simulink model "final_upfc_400kv_wavelet_windfarm_q"  (R2021a)
settings: Solver=VariableStepAuto  StartTime=0.0  StopTime=0.5  RelTol=1e-3
values from neighbouring files (symbols this model uses):
  Ts = 0.00005    (= 5e-05)    [differential_wavelet_with_wind_farm_400.m]
undefined symbols (not defined in the file or in its folder): D11, Delta, DiscIntNeverNeededParam, find_system, level
libraries: powerlib_extras x76, spsThreePhaseVIMeasurementLib x11, simulink_extras x8, spsThreeLevelBridgeLib x8, spsVoltageMeasurementLib x8, spsZigzagPhaseShiftingTransformerLib x8, spsCurrentMeasurementLib x6, spsSeriesRLCBranchLib x5, spsThreePhasePISectionLineLib x5, spsThreePhaseFaultLib x4, spsThreePhaseTransformerTwoWindingsLib x2, spsMultimeterLib x2
(part 7 of 9)

== system final_upfc_400kv_wavelet_windfarm_q/UPFC Controller/SE Control (UPFC)/Firing Pulses Generator/Bridge 1Y /Phase C ==
  note: |
      | |
      | |
      | [Q1]
      | |
      | |
  note: |
      | |
      | [Q2]
      | |
      | |
  note: |
      | |
      | [Q3]
      | |
      | |
  note: |
      | |
      | [G4]
      | |
      | |
      | |
  note: --------[D_NP]---------
  note: --------[D-NN]---------
  note: ---------- A
  note: |
      | |
      | |
      | |
      | |
      | |
      | |
      | |
      | |
      | |
      | |
  note: N -------
  note: - Vdc -------------------------------
  note: + Vdc -------------------------------
  note: Q4,Q1
  note: Q2,Q3
  note: Q1,Q2,Q3,Q4
  note: |
      | |
      | |
      | |
      | |
      | |
      | |
      | |
      | |
      | |
      | |
  note: |
      | |
      | |
      | |
      | |
      | |
      | |
      | |
      | |
      | |
      | |
  note: |
      | |
      | |
      | |
      | |
      | |
      | |
      | |
      | |
      | |
      | |
  note: Pulses timing
      | ===========
  note: Normal 180deg
      | Operation
  note: Normal 180deg
      | Operation
  note: Normal 180deg
      | Operation
  note: I--------------------------------I-----------------------------I--
  note: 0
  note: 180
  note: 360
  note: ******************
  note: ******************
  note: ********************************************
  note: ******************************************
  note: Q1
  note: Q2
  note: Q3
  note: Q4
  note: |
      | |
      | |
  note: |
      | |
      | |
  note: <--Sigma-->
  wt : Inport  PortDimensions=1
  sigma : Inport  Port=2  PortDimensions=1
  D_Alpha : Inport  Port=3  PortDimensions=1
  Constant1 : Constant  Value=[0 -pi]
  Constant2 : Constant  Value=2*pi
  Constant3 : Constant  Value=0
  Constant8 : Constant  Value=pi
  Constant9 : Constant  Value=pi
  Deg->Rad2 : Gain  Gain=0.5  SaturateOnIntegerOverflow=on  OutDataTypeStr=Inherit: Same as input  ParamDataTypeStr=Inherit: Same as input
  Deg->Rad3 : Gain  Gain=-1  SaturateOnIntegerOverflow=on  OutDataTypeStr=Inherit: Same as input  ParamDataTypeStr=Inherit: Same as input
  Gain3 : Gain  Gain=2  SaturateOnIntegerOverflow=on  OutDataTypeStr=Inherit: Same as input  ParamDataTypeStr=Inherit: Same as input
  Logical Operator : Logic
  Logical Operator2 : Logic  Operator=NOT
  Math Function : Math  Operator=mod  SignedPower=on  SaturateOnIntegerOverflow=on
  Mux3 : Mux  Inputs=[2 2]
  Mux4 : Mux  Inputs=2
  Relational Operator : RelationalOperator  RndMeth=Nearest  InputSameDT=on
  Relational Operator1 : RelationalOperator  Operator=<  RndMeth=Nearest  InputSameDT=on
  Selector3 : Selector  InputPortWidth=4  IndexOptions=Index vector (dialog)  Indices=[4 1 2 3]  OutputSizes=1
  Sum{2,4..6} (4 alike) : Sum  InputSameDT=on  SaturateOnIntegerOverflow=on  OutDataTypeStr=Inherit: Same as first input
  Sum3 : Sum  Inputs=+-  InputSameDT=on  SaturateOnIntegerOverflow=on  OutDataTypeStr=Inherit: Same as first input
  Pulses : Outport
  wires:
  Constant1/1 -> Sum2/2
  Constant3/1 -> Relational Operator/2
  Relational Operator/1 -> Logical Operator/1
  Relational Operator1/1 -> Logical Operator/2
  Constant9/1 -> Sum3/1
  sigma/1 -> Sum3/2
  Sum3/1 -> Deg->Rad2/1
  Deg->Rad2/1 -> Sum4/1, Gain3/1  "Beta"
  Constant8/1 -> Sum6/2
  Sum6/1 -> Relational Operator1/2
  Sum2/1 -> Sum4/2
  Sum4/1 -> Math Function/1
  Logical Operator/1 -> Logical Operator2/1, Mux3/1
  Logical Operator2/1 -> Mux3/2
  Mux3/1 -> Selector3/1
  Selector3/1 -> Pulses/1
  Gain3/1 -> Sum6/1
  Math Function/1 -> Relational Operator1/1, Relational Operator/1
  Mux4/1 -> Sum5/2
  Deg->Rad3/1 -> Mux4/2
  D_Alpha/1 -> Deg->Rad3/1, Mux4/1
  wt/1 -> Sum5/1  "wt"
  Sum5/1 -> Sum2/1  "theta"
  Constant2/1 -> Math Function/2

== system final_upfc_400kv_wavelet_windfarm_q/UPFC Controller/SE Control (UPFC)/Firing Pulses Generator/Bridge 2D/Phase A ==
  note: <--Sigma-->
  note: |
      | |
      | |
  note: |
      | |
      | |
  note: Q4
  note: Q3
  note: Q2
  note: Q1
  note: ******************************************
  note: ********************************************
  note: ******************
  note: ******************
  note: 360
  note: 180
  note: 0
  note: I--------------------------------I-----------------------------I--
  note: Normal 180deg
      | Operation
  note: Normal 180deg
      | Operation
  note: Normal 180deg
      | Operation
  note: Pulses timing
      | ===========
  note: |
      | |
      | |
      | |
      | |
      | |
      | |
      | |
      | |
      | |
      | |
  note: |
      | |
      | |
      | |
      | |
      | |
      | |
      | |
      | |
      | |
      | |
  note: |
      | |
      | |
      | |
      | |
      | |
      | |
      | |
      | |
      | |
      | |
  note: Q1,Q2,Q3,Q4
  note: Q2,Q3
  note: Q4,Q1
  note: + Vdc -------------------------------
  note: - Vdc -------------------------------
  note: N -------
  note: |
      | |
      | |
      | |
      | |
      | |
      | |
      | |
      | |
      | |
      | |
  note: ---------- A
  note: --------[D-NN]---------
  note: --------[D_NP]---------
  note: |
      | |
      | [G4]
      | |
      | |
      | |
  note: |
      | |
      | [Q3]
      | |
      | |
  note: |
      | |
      | [Q2]
      | |
      | |
  note: |
      | |
      | |
      | [Q1]
      | |
      | |
  wt : Inport  PortDimensions=1
  sigma : Inport  Port=2  PortDimensions=1
  D_Alpha : Inport  Port=3  PortDimensions=1
  Constant1 : Constant  Value=[0 -pi]
  Constant2 : Constant  Value=2*pi
  Constant3 : Constant  Value=0
  Constant8 : Constant  Value=pi
  Constant9 : Constant  Value=pi
  Deg->Rad2 : Gain  Gain=0.5  SaturateOnIntegerOverflow=on  OutDataTypeStr=Inherit: Same as input  ParamDataTypeStr=Inherit: Same as input
  Deg->Rad3 : Gain  Gain=-1  SaturateOnIntegerOverflow=on  OutDataTypeStr=Inherit: Same as input  ParamDataTypeStr=Inherit: Same as input
  Gain3 : Gain  Gain=2  SaturateOnIntegerOverflow=on  OutDataTypeStr=Inherit: Same as input  ParamDataTypeStr=Inherit: Same as input
  Logical Operator : Logic
  Logical Operator2 : Logic  Operator=NOT
  Math Function : Math  Operator=mod  SignedPower=on  SaturateOnIntegerOverflow=on
  Mux3 : Mux  Inputs=[2 2]
  Mux4 : Mux  Inputs=2
  Relational Operator : RelationalOperator  RndMeth=Nearest  InputSameDT=on
  Relational Operator1 : RelationalOperator  Operator=<  RndMeth=Nearest  InputSameDT=on
  Selector3 : Selector  InputPortWidth=4  IndexOptions=Index vector (dialog)  Indices=[4 1 2 3]  OutputSizes=1
  Sum{2,4..6} (4 alike) : Sum  InputSameDT=on  SaturateOnIntegerOverflow=on  OutDataTypeStr=Inherit: Same as first input
  Sum3 : Sum  Inputs=+-  InputSameDT=on  SaturateOnIntegerOverflow=on  OutDataTypeStr=Inherit: Same as first input
  Pulses : Outport
  wires:
  Constant2/1 -> Math Function/2
  Sum5/1 -> Sum2/1  "theta"
  wt/1 -> Sum5/1  "wt"
  D_Alpha/1 -> Mux4/1, Deg->Rad3/1
  Deg->Rad3/1 -> Mux4/2
  Mux4/1 -> Sum5/2
  Math Function/1 -> Relational Operator/1, Relational Operator1/1
  Gain3/1 -> Sum6/1
  Selector3/1 -> Pulses/1
  Mux3/1 -> Selector3/1
  Logical Operator2/1 -> Mux3/2
  Logical Operator/1 -> Mux3/1, Logical Operator2/1
  Sum4/1 -> Math Function/1
  Sum2/1 -> Sum4/2
  Sum6/1 -> Relational Operator1/2
  Constant8/1 -> Sum6/2
  Deg->Rad2/1 -> Gain3/1, Sum4/1  "Beta"
  Sum3/1 -> Deg->Rad2/1
  sigma/1 -> Sum3/2
  Constant9/1 -> Sum3/1
  Relational Operator1/1 -> Logical Operator/2
  Relational Operator/1 -> Logical Operator/1
  Constant3/1 -> Relational Operator/2
  Constant1/1 -> Sum2/2

== system final_upfc_400kv_wavelet_windfarm_q/UPFC Controller/SE Control (UPFC)/Firing Pulses Generator/Bridge 2D/Phase B ==
  note: |
      | |
      | |
      | [Q1]
      | |
      | |
  note: |
      | |
      | [Q2]
      | |
      | |
  note: |
      | |
      | [Q3]
      | |
      | |
  note: |
      | |
      | [G4]
      | |
      | |
      | |
  note: --------[D_NP]---------
  note: --------[D-NN]---------
  note: ---------- A
  note: |
      | |
      | |
      | |
      | |
      | |
      | |
      | |
      | |
      | |
      | |
  note: N -------
  note: - Vdc -------------------------------
  note: + Vdc -------------------------------
  note: Q4,Q1
  note: Q2,Q3
  note: Q1,Q2,Q3,Q4
  note: |
      | |
      | |
      | |
      | |
      | |
      | |
      | |
      | |
      | |
      | |
  note: |
      | |
      | |
      | |
      | |
      | |
      | |
      | |
      | |
      | |
      | |
  note: |
      | |
      | |
      | |
      | |
      | |
      | |
      | |
      | |
      | |
      | |
  note: Pulses timing
      | ===========
  note: Normal 180deg
      | Operation
  note: Normal 180deg
      | Operation
  note: Normal 180deg
      | Operation
  note: I--------------------------------I-----------------------------I--
  note: 0
  note: 180
  note: 360
  note: ******************
  note: ******************
  note: ********************************************
  note: ******************************************
  note: Q1
  note: Q2
  note: Q3
  note: Q4
  note: |
      | |
      | |
  note: |
      | |
      | |
  note: <--Sigma-->
  wt : Inport  PortDimensions=1
  sigma : Inport  Port=2  PortDimensions=1
  D_Alpha : Inport  Port=3  PortDimensions=1
  Constant1 : Constant  Value=[0 -pi]
  Constant2 : Constant  Value=2*pi
  Constant3 : Constant  Value=0
  Constant8 : Constant  Value=pi
  Constant9 : Constant  Value=pi
  Deg->Rad2 : Gain  Gain=0.5  SaturateOnIntegerOverflow=on  OutDataTypeStr=Inherit: Same as input  ParamDataTypeStr=Inherit: Same as input
  Deg->Rad3 : Gain  Gain=-1  SaturateOnIntegerOverflow=on  OutDataTypeStr=Inherit: Same as input  ParamDataTypeStr=Inherit: Same as input
  Gain3 : Gain  Gain=2  SaturateOnIntegerOverflow=on  OutDataTypeStr=Inherit: Same as input  ParamDataTypeStr=Inherit: Same as input
  Logical Operator : Logic
  Logical Operator2 : Logic  Operator=NOT
  Math Function : Math  Operator=mod  SignedPower=on  SaturateOnIntegerOverflow=on
  Mux3 : Mux  Inputs=[2 2]
  Mux4 : Mux  Inputs=2
  Relational Operator : RelationalOperator  RndMeth=Nearest  InputSameDT=on
  Relational Operator1 : RelationalOperator  Operator=<  RndMeth=Nearest  InputSameDT=on
  Selector3 : Selector  InputPortWidth=4  IndexOptions=Index vector (dialog)  Indices=[4 1 2 3]  OutputSizes=1
  Sum{2,4..6} (4 alike) : Sum  InputSameDT=on  SaturateOnIntegerOverflow=on  OutDataTypeStr=Inherit: Same as first input
  Sum3 : Sum  Inputs=+-  InputSameDT=on  SaturateOnIntegerOverflow=on  OutDataTypeStr=Inherit: Same as first input
  Pulses : Outport
  wires:
  Constant1/1 -> Sum2/2
  Constant3/1 -> Relational Operator/2
  Relational Operator/1 -> Logical Operator/1
  Relational Operator1/1 -> Logical Operator/2
  Constant9/1 -> Sum3/1
  sigma/1 -> Sum3/2
  Sum3/1 -> Deg->Rad2/1
  Deg->Rad2/1 -> Sum4/1, Gain3/1  "Beta"
  Constant8/1 -> Sum6/2
  Sum6/1 -> Relational Operator1/2
  Sum2/1 -> Sum4/2
  Sum4/1 -> Math Function/1
  Logical Operator/1 -> Logical Operator2/1, Mux3/1
  Logical Operator2/1 -> Mux3/2
  Mux3/1 -> Selector3/1
  Selector3/1 -> Pulses/1
  Gain3/1 -> Sum6/1
  Math Function/1 -> Relational Operator1/1, Relational Operator/1
  Mux4/1 -> Sum5/2
  Deg->Rad3/1 -> Mux4/2
  D_Alpha/1 -> Deg->Rad3/1, Mux4/1
  wt/1 -> Sum5/1  "wt"
  Sum5/1 -> Sum2/1  "theta"
  Constant2/1 -> Math Function/2

== system final_upfc_400kv_wavelet_windfarm_q/UPFC Controller/SE Control (UPFC)/Firing Pulses Generator/Bridge 2D/Phase C ==
  note: <--Sigma-->
  note: |
      | |
      | |
  note: |
      | |
      | |
  note: Q4
  note: Q3
  note: Q2
  note: Q1
  note: ******************************************
  note: ********************************************
  note: ******************
  note: ******************
  note: 360
  note: 180
  note: 0
  note: I--------------------------------I-----------------------------I--
  note: Normal 180deg
      | Operation
  note: Normal 180deg
      | Operation
  note: Normal 180deg
      | Operation
  note: Pulses timing
      | ===========
  note: |
      | |
      | |
      | |
      | |
      | |
      | |
      | |
      | |
      | |
      | |
  note: |
      | |
      | |
      | |
      | |
      | |
      | |
      | |
      | |
      | |
      | |
  note: |
      | |
      | |
      | |
      | |
      | |
      | |
      | |
      | |
      | |
      | |
  note: Q1,Q2,Q3,Q4
  note: Q2,Q3
  note: Q4,Q1
  note: + Vdc -------------------------------
  note: - Vdc -------------------------------
  note: N -------
  note: |
      | |
      | |
      | |
      | |
      | |
      | |
      | |
      | |
      | |
      | |
  note: ---------- A
  note: --------[D-NN]---------
  note: --------[D_NP]---------
  note: |
      | |
      | [G4]
      | |
      | |
      | |
  note: |
      | |
      | [Q3]
      | |
      | |
  note: |
      | |
      | [Q2]
      | |
      | |
  note: |
      | |
      | |
      | [Q1]
      | |
      | |
  wt : Inport  PortDimensions=1
  sigma : Inport  Port=2  PortDimensions=1
  D_Alpha : Inport  Port=3  PortDimensions=1
  Constant1 : Constant  Value=[0 -pi]
  Constant2 : Constant  Value=2*pi
  Constant3 : Constant  Value=0
  Constant8 : Constant  Value=pi
  Constant9 : Constant  Value=pi
  Deg->Rad2 : Gain  Gain=0.5  SaturateOnIntegerOverflow=on  OutDataTypeStr=Inherit: Same as input  ParamDataTypeStr=Inherit: Same as input
  Deg->Rad3 : Gain  Gain=-1  SaturateOnIntegerOverflow=on  OutDataTypeStr=Inherit: Same as input  ParamDataTypeStr=Inherit: Same as input
  Gain3 : Gain  Gain=2  SaturateOnIntegerOverflow=on  OutDataTypeStr=Inherit: Same as input  ParamDataTypeStr=Inherit: Same as input
  Logical Operator : Logic
  Logical Operator2 : Logic  Operator=NOT
  Math Function : Math  Operator=mod  SignedPower=on  SaturateOnIntegerOverflow=on
  Mux3 : Mux  Inputs=[2 2]
  Mux4 : Mux  Inputs=2
  Relational Operator : RelationalOperator  RndMeth=Nearest  InputSameDT=on
  Relational Operator1 : RelationalOperator  Operator=<  RndMeth=Nearest  InputSameDT=on
  Selector3 : Selector  InputPortWidth=4  IndexOptions=Index vector (dialog)  Indices=[4 1 2 3]  OutputSizes=1
  Sum{2,4..6} (4 alike) : Sum  InputSameDT=on  SaturateOnIntegerOverflow=on  OutDataTypeStr=Inherit: Same as first input
  Sum3 : Sum  Inputs=+-  InputSameDT=on  SaturateOnIntegerOverflow=on  OutDataTypeStr=Inherit: Same as first input
  Pulses : Outport
  wires:
  Constant2/1 -> Math Function/2
  Sum5/1 -> Sum2/1  "theta"
  wt/1 -> Sum5/1  "wt"
  D_Alpha/1 -> Mux4/1, Deg->Rad3/1
  Deg->Rad3/1 -> Mux4/2
  Mux4/1 -> Sum5/2
  Math Function/1 -> Relational Operator/1, Relational Operator1/1
  Gain3/1 -> Sum6/1
  Selector3/1 -> Pulses/1
  Mux3/1 -> Selector3/1
  Logical Operator2/1 -> Mux3/2
  Logical Operator/1 -> Mux3/1, Logical Operator2/1
  Sum4/1 -> Math Function/1
  Sum2/1 -> Sum4/2
  Sum6/1 -> Relational Operator1/2
  Constant8/1 -> Sum6/2
  Deg->Rad2/1 -> Gain3/1, Sum4/1  "Beta"
  Sum3/1 -> Deg->Rad2/1
  sigma/1 -> Sum3/2
  Constant9/1 -> Sum3/1
  Relational Operator1/1 -> Logical Operator/2
  Relational Operator/1 -> Logical Operator/1
  Constant3/1 -> Relational Operator/2
  Constant1/1 -> Sum2/2

== system final_upfc_400kv_wavelet_windfarm_q/UPFC Controller/SE Control (UPFC)/Firing Pulses Generator/Bridge 2Y/Phase A ==
  note: |
      | |
      | |
      | [Q1]
      | |
      | |
  note: |
      | |
      | [Q2]
      | |
      | |
  note: |
      | |
      | [Q3]
      | |
      | |
  note: |
      | |
      | [G4]
      | |
      | |
      | |
  note: --------[D_NP]---------
  note: --------[D-NN]---------
  note: ---------- A
  note: |
      | |
      | |
      | |
      | |
      | |
      | |
      | |
      | |
      | |
      | |
  note: N -------
  note: - Vdc -------------------------------
  note: + Vdc -------------------------------
  note: Q4,Q1
  note: Q2,Q3
  note: Q1,Q2,Q3,Q4
  note: |
      | |
      | |
      | |
      | |
      | |
      | |
      | |
      | |
      | |
      | |
  note: |
      | |
      | |
      | |
      | |
      | |
      | |
      | |
      | |
      | |
      | |
  note: |
      | |
      | |
      | |
      | |
      | |
      | |
      | |
      | |
      | |
      | |
  note: Pulses timing
      | ===========
  note: Normal 180deg
      | Operation
  note: Normal 180deg
      | Operation
  note: Normal 180deg
      | Operation
  note: I--------------------------------I-----------------------------I--
  note: 0
  note: 180
  note: 360
  note: ******************
  note: ******************
  note: ********************************************
  note: ******************************************
  note: Q1
  note: Q2
  note: Q3
  note: Q4
  note: |
      | |
      | |
  note: |
      | |
      | |
  note: <--Sigma-->
  wt : Inport  PortDimensions=1
  sigma : Inport  Port=2  PortDimensions=1
  D_Alpha : Inport  Port=3  PortDimensions=1
  Constant1 : Constant  Value=[0 -pi]
  Constant2 : Constant  Value=2*pi
  Constant3 : Constant  Value=0
  Constant8 : Constant  Value=pi
  Constant9 : Constant  Value=pi
  Deg->Rad2 : Gain  Gain=0.5  SaturateOnIntegerOverflow=on  OutDataTypeStr=Inherit: Same as input  ParamDataTypeStr=Inherit: Same as input
  Deg->Rad3 : Gain  Gain=-1  SaturateOnIntegerOverflow=on  OutDataTypeStr=Inherit: Same as input  ParamDataTypeStr=Inherit: Same as input
  Gain3 : Gain  Gain=2  SaturateOnIntegerOverflow=on  OutDataTypeStr=Inherit: Same as input  ParamDataTypeStr=Inherit: Same as input
  Logical Operator : Logic
  Logical Operator2 : Logic  Operator=NOT
  Math Function : Math  Operator=mod  SignedPower=on  SaturateOnIntegerOverflow=on
  Mux3 : Mux  Inputs=[2 2]
  Mux4 : Mux  Inputs=2
  Relational Operator : RelationalOperator  RndMeth=Nearest  InputSameDT=on
  Relational Operator1 : RelationalOperator  Operator=<  RndMeth=Nearest  InputSameDT=on
  Selector3 : Selector  InputPortWidth=4  IndexOptions=Index vector (dialog)  Indices=[4 1 2 3]  OutputSizes=1
  Sum{2,4..6} (4 alike) : Sum  InputSameDT=on  SaturateOnIntegerOverflow=on  OutDataTypeStr=Inherit: Same as first input
  Sum3 : Sum  Inputs=+-  InputSameDT=on  SaturateOnIntegerOverflow=on  OutDataTypeStr=Inherit: Same as first input
  Pulses : Outport
  wires:
  Constant1/1 -> Sum2/2
  Constant3/1 -> Relational Operator/2
  Relational Operator/1 -> Logical Operator/1
  Relational Operator1/1 -> Logical Operator/2
  Constant9/1 -> Sum3/1
  sigma/1 -> Sum3/2
  Sum3/1 -> Deg->Rad2/1
  Deg->Rad2/1 -> Sum4/1, Gain3/1  "Beta"
  Constant8/1 -> Sum6/2
  Sum6/1 -> Relational Operator1/2
  Sum2/1 -> Sum4/2
  Sum4/1 -> Math Function/1
  Logical Operator/1 -> Logical Operator2/1, Mux3/1
  Logical Operator2/1 -> Mux3/2
  Mux3/1 -> Selector3/1
  Selector3/1 -> Pulses/1
  Gain3/1 -> Sum6/1
  Math Function/1 -> Relational Operator1/1, Relational Operator/1
  Mux4/1 -> Sum5/2
  Deg->Rad3/1 -> Mux4/2
  D_Alpha/1 -> Deg->Rad3/1, Mux4/1
  wt/1 -> Sum5/1  "wt"
  Sum5/1 -> Sum2/1  "theta"
  Constant2/1 -> Math Function/2

== system final_upfc_400kv_wavelet_windfarm_q/UPFC Controller/SE Control (UPFC)/Firing Pulses Generator/Bridge 2Y/Phase B ==
  note: <--Sigma-->
  note: |
      | |
      | |
  note: |
      | |
      | |
  note: Q4
  note: Q3
  note: Q2
  note: Q1
  note: ******************************************
  note: ********************************************
  note: ******************
  note: ******************
  note: 360
  note: 180
  note: 0
  note: I--------------------------------I-----------------------------I--
  note: Normal 180deg
      | Operation
  note: Normal 180deg
      | Operation
  note: Normal 180deg
      | Operation
  note: Pulses timing
      | ===========
  note: |
      | |
      | |
      | |
      | |
      | |
      | |
      | |
      | |
      | |
      | |
  note: |
      | |
      | |
      | |
      | |
      | |
      | |
      | |
      | |
      | |
      | |
  note: |
      | |
      | |
      | |
      | |
      | |
      | |
      | |
      | |
      | |
      | |
  note: Q1,Q2,Q3,Q4
  note: Q2,Q3
  note: Q4,Q1
  note: + Vdc -------------------------------
  note: - Vdc -------------------------------
  note: N -------
  note: |
      | |
      | |
      | |
      | |
      | |
      | |
      | |
      | |
      | |
      | |
  note: ---------- A
  note: --------[D-NN]---------
  note: --------[D_NP]---------
  note: |
      | |
      | [G4]
      | |
      | |
      | |
  note: |
      | |
      | [Q3]
      | |
      | |
  note: |
      | |
      | [Q2]
      | |
      | |
  note: |
      | |
      | |
      | [Q1]
      | |
      | |
  wt : Inport  PortDimensions=1
  sigma : Inport  Port=2  PortDimensions=1
  D_Alpha : Inport  Port=3  PortDimensions=1
  Constant1 : Constant  Value=[0 -pi]
  Constant2 : Constant  Value=2*pi
  Constant3 : Constant  Value=0
  Constant8 : Constant  Value=pi
  Constant9 : Constant  Value=pi
  Deg->Rad2 : Gain  Gain=0.5  SaturateOnIntegerOverflow=on  OutDataTypeStr=Inherit: Same as input  ParamDataTypeStr=Inherit: Same as input
  Deg->Rad3 : Gain  Gain=-1  SaturateOnIntegerOverflow=on  OutDataTypeStr=Inherit: Same as input  ParamDataTypeStr=Inherit: Same as input
  Gain3 : Gain  Gain=2  SaturateOnIntegerOverflow=on  OutDataTypeStr=Inherit: Same as input  ParamDataTypeStr=Inherit: Same as input
  Logical Operator : Logic
  Logical Operator2 : Logic  Operator=NOT
  Math Function : Math  Operator=mod  SignedPower=on  SaturateOnIntegerOverflow=on
  Mux3 : Mux  Inputs=[2 2]
  Mux4 : Mux  Inputs=2
  Relational Operator : RelationalOperator  RndMeth=Nearest  InputSameDT=on
  Relational Operator1 : RelationalOperator  Operator=<  RndMeth=Nearest  InputSameDT=on
  Selector3 : Selector  InputPortWidth=4  IndexOptions=Index vector (dialog)  Indices=[4 1 2 3]  OutputSizes=1
  Sum{2,4..6} (4 alike) : Sum  InputSameDT=on  SaturateOnIntegerOverflow=on  OutDataTypeStr=Inherit: Same as first input
  Sum3 : Sum  Inputs=+-  InputSameDT=on  SaturateOnIntegerOverflow=on  OutDataTypeStr=Inherit: Same as first input
  Pulses : Outport
  wires:
  Constant2/1 -> Math Function/2
  Sum5/1 -> Sum2/1  "theta"
  wt/1 -> Sum5/1  "wt"
  D_Alpha/1 -> Mux4/1, Deg->Rad3/1
  Deg->Rad3/1 -> Mux4/2
  Mux4/1 -> Sum5/2
  Math Function/1 -> Relational Operator/1, Relational Operator1/1
  Gain3/1 -> Sum6/1
  Selector3/1 -> Pulses/1
  Mux3/1 -> Selector3/1
  Logical Operator2/1 -> Mux3/2
  Logical Operator/1 -> Mux3/1, Logical Operator2/1
  Sum4/1 -> Math Function/1
  Sum2/1 -> Sum4/2
  Sum6/1 -> Relational Operator1/2
  Constant8/1 -> Sum6/2
  Deg->Rad2/1 -> Gain3/1, Sum4/1  "Beta"
  Sum3/1 -> Deg->Rad2/1
  sigma/1 -> Sum3/2
  Constant9/1 -> Sum3/1
  Relational Operator1/1 -> Logical Operator/2
  Relational Operator/1 -> Logical Operator/1
  Constant3/1 -> Relational Operator/2
  Constant1/1 -> Sum2/2

== system final_upfc_400kv_wavelet_windfarm_q/UPFC Controller/SE Control (UPFC)/Firing Pulses Generator/Bridge 2Y/Phase C ==
  note: |
      | |
      | |
      | [Q1]
      | |
      | |
  note: |
      | |
      | [Q2]
      | |
      | |
  note: |
      | |
      | [Q3]
      | |
      | |
  note: |
      | |
      | [G4]
      | |
      | |
      | |
  note: --------[D_NP]---------
  note: --------[D-NN]---------
  note: ---------- A
  note: |
      | |
      | |
      | |
      | |
      | |
      | |
      | |
      | |
      | |
      | |
  note: N -------
  note: - Vdc -------------------------------
  note: + Vdc -------------------------------
  note: Q4,Q1
  note: Q2,Q3
  note: Q1,Q2,Q3,Q4
  note: |
      | |
      | |
      | |
      | |
      | |
      | |
      | |
      | |
      | |
      | |
  note: |
      | |
      | |
      | |
      | |
      | |
      | |
      | |
      | |
      | |
      | |
  note: |
      | |
      | |
      | |
      | |
      | |
      | |
      | |
      | |
      | |
      | |
  note: Pulses timing
      | ===========
  note: Normal 180deg
      | Operation
  note: Normal 180deg
      | Operation
  note: Normal 180deg
      | Operation
  note: I--------------------------------I-----------------------------I--
  note: 0
  note: 180
  note: 360
  note: ******************
  note: ******************
  note: ********************************************
  note: ******************************************
  note: Q1
  note: Q2
  note: Q3
  note: Q4
  note: |
      | |
      | |
  note: |
      | |
      | |
  note: <--Sigma-->
  wt : Inport  PortDimensions=1
  sigma : Inport  Port=2  PortDimensions=1
  D_Alpha : Inport  Port=3  PortDimensions=1
  Constant1 : Constant  Value=[0 -pi]
  Constant2 : Constant  Value=2*pi
  Constant3 : Constant  Value=0
  Constant8 : Constant  Value=pi
  Constant9 : Constant  Value=pi
  Deg->Rad2 : Gain  Gain=0.5  SaturateOnIntegerOverflow=on  OutDataTypeStr=Inherit: Same as input  ParamDataTypeStr=Inherit: Same as input
  Deg->Rad3 : Gain  Gain=-1  SaturateOnIntegerOverflow=on  OutDataTypeStr=Inherit: Same as input  ParamDataTypeStr=Inherit: Same as input
  Gain3 : Gain  Gain=2  SaturateOnIntegerOverflow=on  OutDataTypeStr=Inherit: Same as input  ParamDataTypeStr=Inherit: Same as input
  Logical Operator : Logic
  Logical Operator2 : Logic  Operator=NOT
  Math Function : Math  Operator=mod  SignedPower=on  SaturateOnIntegerOverflow=on
  Mux3 : Mux  Inputs=[2 2]
  Mux4 : Mux  Inputs=2
  Relational Operator : RelationalOperator  RndMeth=Nearest  InputSameDT=on
  Relational Operator1 : RelationalOperator  Operator=<  RndMeth=Nearest  InputSameDT=on
  Selector3 : Selector  InputPortWidth=4  IndexOptions=Index vector (dialog)  Indices=[4 1 2 3]  OutputSizes=1
  Sum{2,4..6} (4 alike) : Sum  InputSameDT=on  SaturateOnIntegerOverflow=on  OutDataTypeStr=Inherit: Same as first input
  Sum3 : Sum  Inputs=+-  InputSameDT=on  SaturateOnIntegerOverflow=on  OutDataTypeStr=Inherit: Same as first input
  Pulses : Outport
  wires:
  Constant1/1 -> Sum2/2
  Constant3/1 -> Relational Operator/2
  Relational Operator/1 -> Logical Operator/1
  Relational Operator1/1 -> Logical Operator/2
  Constant9/1 -> Sum3/1
  sigma/1 -> Sum3/2
  Sum3/1 -> Deg->Rad2/1
  Deg->Rad2/1 -> Sum4/1, Gain3/1  "Beta"
  Constant8/1 -> Sum6/2
  Sum6/1 -> Relational Operator1/2
  Sum2/1 -> Sum4/2
  Sum4/1 -> Math Function/1
  Logical Operator/1 -> Logical Operator2/1, Mux3/1
  Logical Operator2/1 -> Mux3/2
  Mux3/1 -> Selector3/1
  Selector3/1 -> Pulses/1
  Gain3/1 -> Sum6/1
  Math Function/1 -> Relational Operator1/1, Relational Operator/1
  Mux4/1 -> Sum5/2
  Deg->Rad3/1 -> Mux4/2
  D_Alpha/1 -> Deg->Rad3/1, Mux4/1
  wt/1 -> Sum5/1  "wt"
  Sum5/1 -> Sum2/1  "theta"
  Constant2/1 -> Math Function/2

== system final_upfc_400kv_wavelet_windfarm_q/UPFC Controller/SE Control (UPFC)/Measurement System/Voltage Measurement/Discrete Variable Frequency Mean value1 ==
  note: Pierre Giroux, Gilbert Sybille
      | Power System Simulation Laboratory
      | IREQ, Hydro-Quebc
  note: Variable frequency - Discrete Mean Value
  Freq : Inport
  In : Inport  Port=2
  Constant : Constant  Value=Vinit
  Gain : Gain  Gain=Ts  SaturateOnIntegerOverflow=on  OutDataTypeStr=Inherit: Same as input  ParamDataTypeStr=Inherit: Same as input
  Integ4 : DiscreteIntegrator  IntegratorMethod=Integration: Trapezoidal  SampleTime=Ts  ICPrevOutput=DiscIntNeverNeededParam  ICPrevScaledInput=DiscIntNeverNeededParam
  K2 : Constant  Value=Ts/2
  Number of sample/cycle : Fcn  Expr=1/(u[1]+1e-6)/Ts
  Product : Product  InputSameDT=on  SaturateOnIntegerOverflow=on  OutDataTypeStr=Inherit: Same as first input
  Product1 : Product  Inputs=*/*  InputSameDT=on  SaturateOnIntegerOverflow=on  OutDataTypeStr=Inherit: Same as first input
  Rounding Function : Rounding  Operator=round
  Step : Step  Time=1/Finit  SampleTime=Ts
  Sum3 : Sum  Inputs=-+  InputSameDT=on  SaturateOnIntegerOverflow=on  OutDataTypeStr=Inherit: Same as first input
  Sum4 : Sum  Inputs=-+  InputSameDT=on  SaturateOnIntegerOverflow=on  OutDataTypeStr=Inherit: Same as first input
  Sum5 : Sum  InputSameDT=on  SaturateOnIntegerOverflow=on  OutDataTypeStr=Inherit: Same as first input
  Sum7 : Sum  Inputs=-+  InputSameDT=on  SaturateOnIntegerOverflow=on  OutDataTypeStr=Inherit: Same as first input
  Switch : Switch  Threshold=0.5  SaturateOnIntegerOverflow=on  InputSameDT=on
  Variable Transport Delay2 : VariableTransportDelay  MaximumDelay=20e-3
  Mean : Outport
  wires:
  Product1/1 -> Sum5/2  "Correction"
  In/1 -> Product1/3, Integ4/1  "In"
  Product/1 -> Sum5/1  "Mean value"
  Variable Transport Delay2/1 -> Sum7/1
  Sum7/1 -> Product/1
  Integ4/1 -> Variable Transport Delay2/1, Sum7/2
  Freq/1 -> Product/2, Number of sample/cycle/1  "Freq"
  K2/1 -> Sum3/1
  Gain/1 -> Sum3/2
  Rounding Function/1 -> Gain/1, Product1/2, Sum4/1
  Sum4/1 -> Product1/1
  Number of sample/cycle/1 -> Rounding Function/1, Sum4/2
  Sum3/1 -> Variable Transport Delay2/2  "Delay"
  Sum5/1 -> Switch/1
  Step/1 -> Switch/2
  Constant/1 -> Switch/3
  Switch/1 -> Mean/1

== system final_upfc_400kv_wavelet_windfarm_q/UPFC Controller/SE Control (UPFC)/Measurement System/Voltage Measurement/Discrete Variable Frequency Mean value2 ==
  note: Pierre Giroux, Gilbert Sybille
      | Power System Simulation Laboratory
      | IREQ, Hydro-Quebc
  note: Variable frequency - Discrete Mean Value
  Freq : Inport
  In : Inport  Port=2
  Constant : Constant  Value=Vinit
  Gain : Gain  Gain=Ts  SaturateOnIntegerOverflow=on  OutDataTypeStr=Inherit: Same as input  ParamDataTypeStr=Inherit: Same as input
  Integ4 : DiscreteIntegrator  IntegratorMethod=Integration: Trapezoidal  SampleTime=Ts  ICPrevOutput=DiscIntNeverNeededParam  ICPrevScaledInput=DiscIntNeverNeededParam
  K2 : Constant  Value=Ts/2
  Number of sample/cycle : Fcn  Expr=1/(u[1]+1e-6)/Ts
  Product : Product  InputSameDT=on  SaturateOnIntegerOverflow=on  OutDataTypeStr=Inherit: Same as first input
  Product1 : Product  Inputs=*/*  InputSameDT=on  SaturateOnIntegerOverflow=on  OutDataTypeStr=Inherit: Same as first input
  Rounding Function : Rounding  Operator=round
  Step : Step  Time=1/Finit  SampleTime=Ts
  Sum3 : Sum  Inputs=-+  InputSameDT=on  SaturateOnIntegerOverflow=on  OutDataTypeStr=Inherit: Same as first input
  Sum4 : Sum  Inputs=-+  InputSameDT=on  SaturateOnIntegerOverflow=on  OutDataTypeStr=Inherit: Same as first input
  Sum5 : Sum  InputSameDT=on  SaturateOnIntegerOverflow=on  OutDataTypeStr=Inherit: Same as first input
  Sum7 : Sum  Inputs=-+  InputSameDT=on  SaturateOnIntegerOverflow=on  OutDataTypeStr=Inherit: Same as first input
  Switch : Switch  Threshold=0.5  SaturateOnIntegerOverflow=on  InputSameDT=on
  Variable Transport Delay2 : VariableTransportDelay  MaximumDelay=20e-3
  Mean : Outport
  wires:
  Product1/1 -> Sum5/2  "Correction"
  In/1 -> Product1/3, Integ4/1  "In"
  Product/1 -> Sum5/1  "Mean value"
  Variable Transport Delay2/1 -> Sum7/1
  Sum7/1 -> Product/1
  Integ4/1 -> Variable Transport Delay2/1, Sum7/2
  Freq/1 -> Product/2, Number of sample/cycle/1  "Freq"
  K2/1 -> Sum3/1
  Gain/1 -> Sum3/2
  Rounding Function/1 -> Gain/1, Product1/2, Sum4/1
  Sum4/1 -> Product1/1
  Number of sample/cycle/1 -> Rounding Function/1, Sum4/2
  Sum3/1 -> Variable Transport Delay2/2  "Delay"
  Sum5/1 -> Switch/1
  Step/1 -> Switch/2
  Constant/1 -> Switch/3
  Switch/1 -> Mean/1

== system final_upfc_400kv_wavelet_windfarm_q/UPFC Controller/SE Control (UPFC)/Measurement System/Voltage Measurement1/Discrete Variable Frequency Mean value1 ==
  note: Variable frequency - Discrete Mean Value
  note: Pierre Giroux, Gilbert Sybille
      | Power System Simulation Laboratory
      | IREQ, Hydro-Quebc
  Freq : Inport
  In : Inport  Port=2
  Constant : Constant  Value=Vinit
  Gain : Gain  Gain=Ts  SaturateOnIntegerOverflow=on  OutDataTypeStr=Inherit: Same as input  ParamDataTypeStr=Inherit: Same as input
  Integ4 : DiscreteIntegrator  IntegratorMethod=Integration: Trapezoidal  SampleTime=Ts  ICPrevOutput=DiscIntNeverNeededParam  ICPrevScaledInput=DiscIntNeverNeededParam
  K2 : Constant  Value=Ts/2
  Number of sample/cycle : Fcn  Expr=1/(u[1]+1e-6)/Ts
  Product : Product  InputSameDT=on  SaturateOnIntegerOverflow=on  OutDataTypeStr=Inherit: Same as first input
  Product1 : Product  Inputs=*/*  InputSameDT=on  SaturateOnIntegerOverflow=on  OutDataTypeStr=Inherit: Same as first input
  Rounding Function : Rounding  Operator=round
  Step : Step  Time=1/Finit  SampleTime=Ts
  Sum3 : Sum  Inputs=-+  InputSameDT=on  SaturateOnIntegerOverflow=on  OutDataTypeStr=Inherit: Same as first input
  Sum4 : Sum  Inputs=-+  InputSameDT=on  SaturateOnIntegerOverflow=on  OutDataTypeStr=Inherit: Same as first input
  Sum5 : Sum  InputSameDT=on  SaturateOnIntegerOverflow=on  OutDataTypeStr=Inherit: Same as first input
  Sum7 : Sum  Inputs=-+  InputSameDT=on  SaturateOnIntegerOverflow=on  OutDataTypeStr=Inherit: Same as first input
  Switch : Switch  Threshold=0.5  SaturateOnIntegerOverflow=on  InputSameDT=on
  Variable Transport Delay2 : VariableTransportDelay  MaximumDelay=20e-3
  Mean : Outport
  wires:
  Switch/1 -> Mean/1
  Constant/1 -> Switch/3
  Step/1 -> Switch/2
  Sum5/1 -> Switch/1
  Sum3/1 -> Variable Transport Delay2/2  "Delay"
  Number of sample/cycle/1 -> Sum4/2, Rounding Function/1
  Sum4/1 -> Product1/1
  Rounding Function/1 -> Sum4/1, Product1/2, Gain/1
  Gain/1 -> Sum3/2
  K2/1 -> Sum3/1
  Freq/1 -> Number of sample/cycle/1, Product/2  "Freq"
  Integ4/1 -> Sum7/2, Variable Transport Delay2/1
  Sum7/1 -> Product/1
  Variable Transport Delay2/1 -> Sum7/1
  Product/1 -> Sum5/1  "Mean value"
  In/1 -> Integ4/1, Product1/3  "In"
  Product1/1 -> Sum5/2  "Correction"

== system final_upfc_400kv_wavelet_windfarm_q/UPFC Controller/SE Control (UPFC)/Measurement System/Voltage Measurement1/Discrete Variable Frequency Mean value2 ==
  note: Variable frequency - Discrete Mean Value
  note: Pierre Giroux, Gilbert Sybille
      | Power System Simulation Laboratory
      | IREQ, Hydro-Quebc
  Freq : Inport
  In : Inport  Port=2
  Constant : Constant  Value=Vinit
  Gain : Gain  Gain=Ts  SaturateOnIntegerOverflow=on  OutDataTypeStr=Inherit: Same as input  ParamDataTypeStr=Inherit: Same as input
  Integ4 : DiscreteIntegrator  IntegratorMethod=Integration: Trapezoidal  SampleTime=Ts  ICPrevOutput=DiscIntNeverNeededParam  ICPrevScaledInput=DiscIntNeverNeededParam
  K2 : Constant  Value=Ts/2
  Number of sample/cycle : Fcn  Expr=1/(u[1]+1e-6)/Ts
  Product : Product  InputSameDT=on  SaturateOnIntegerOverflow=on  OutDataTypeStr=Inherit: Same as first input
  Product1 : Product  Inputs=*/*  InputSameDT=on  SaturateOnIntegerOverflow=on  OutDataTypeStr=Inherit: Same as first input
  Rounding Function : Rounding  Operator=round
  Step : Step  Time=1/Finit  SampleTime=Ts
  Sum3 : Sum  Inputs=-+  InputSameDT=on  SaturateOnIntegerOverflow=on  OutDataTypeStr=Inherit: Same as first input
  Sum4 : Sum  Inputs=-+  InputSameDT=on  SaturateOnIntegerOverflow=on  OutDataTypeStr=Inherit: Same as first input
  Sum5 : Sum  InputSameDT=on  SaturateOnIntegerOverflow=on  OutDataTypeStr=Inherit: Same as first input
  Sum7 : Sum  Inputs=-+  InputSameDT=on  SaturateOnIntegerOverflow=on  OutDataTypeStr=Inherit: Same as first input
  Switch : Switch  Threshold=0.5  SaturateOnIntegerOverflow=on  InputSameDT=on
  Variable Transport Delay2 : VariableTransportDelay  MaximumDelay=20e-3
  Mean : Outport
  wires:
  Switch/1 -> Mean/1
  Constant/1 -> Switch/3
  Step/1 -> Switch/2
  Sum5/1 -> Switch/1
  Sum3/1 -> Variable Transport Delay2/2  "Delay"
  Number of sample/cycle/1 -> Sum4/2, Rounding Function/1
  Sum4/1 -> Product1/1
  Rounding Function/1 -> Sum4/1, Product1/2, Gain/1
  Gain/1 -> Sum3/2
  K2/1 -> Sum3/1
  Freq/1 -> Number of sample/cycle/1, Product/2  "Freq"
  Integ4/1 -> Sum7/2, Variable Transport Delay2/1
  Sum7/1 -> Product/1
  Variable Transport Delay2/1 -> Sum7/1
  Product/1 -> Sum5/1  "Mean value"
  In/1 -> Integ4/1, Product1/3  "In"
  Product1/1 -> Sum5/2  "Correction"

== system final_upfc_400kv_wavelet_windfarm_q/UPFC Controller/SE Control (UPFC)/Vd,Vq Selection (Auto//Man) and Limit Computation/Vd,Vq Selection and Limit Computation/Vd,Vq Limit Computation ==
  note: Mag = sqrt( Vd^2 + Vq^2 )
  note: If Mag > Mag_Limit :
  note: Vd=Mag_Limit / Mag * Vd*
  note: Vq=Mag_Limit / Mag * Vq*
  VdVq* : Inport  PortDimensions=2
  Avoid div 0 : Saturate  UpperLimit=1e6  LowerLimit=1e-6
  Demux : Demux  Outputs=2
      settings: DisplayOption=none
  Mag_Limit : Constant  Value=0.105
  Math Function1 : Math  Operator=hypot  SignedPower=on  SaturateOnIntegerOverflow=on
  Product2 : Product  Inputs=*/  InputSameDT=on  SaturateOnIntegerOverflow=on  OutDataTypeStr=Inherit: Same as first input
  Product3 : Product  InputSameDT=on  SaturateOnIntegerOverflow=on  OutDataTypeStr=Inherit: Same as first input
  Relational Operator2 : RelationalOperator  Operator=>  RndMeth=Nearest  InputSameDT=on
  Switch2 : Switch  Threshold=0.5  SaturateOnIntegerOverflow=on  InputSameDT=on
  VdVq : Outport
  wires:
  VdVq*/1 -> Switch2/3, Product3/1, Demux/1
  Relational Operator2/1 -> Switch2/2
  Mag_Limit/1 -> Relational Operator2/2, Product2/1
  Switch2/1 -> VdVq/1
  Product3/1 -> Switch2/1
  Product2/1 -> Product3/2
  Demux/1 -> Math Function1/1
  Demux/2 -> Math Function1/2
  Math Function1/1 -> Relational Operator2/1, Avoid div 0/1
  Avoid div 0/1 -> Product2/2

== system final_upfc_400kv_wavelet_windfarm_q/UPFC Controller/SH Control (STATCOM)/Firing Pulses Generator/Bridge 1D/Phase A ==
  note: <--Sigma-->
  note: |
      | |
      | |
  note: |
      | |
      | |
  note: Q4
  note: Q3
  note: Q2
  note: Q1
  note: ******************************************
  note: ********************************************
  note: ******************
  note: ******************
  note: 360
  note: 180
  note: 0
  note: I--------------------------------I-----------------------------I--
  note: Normal 180deg
      | Operation
  note: Normal 180deg
      | Operation
  note: Normal 180deg
      | Operation
  note: Pulses timing
      | ===========
  note: |
      | |
      | |
      | |
      | |
      | |
      | |
      | |
      | |
      | |
      | |
  note: |
      | |
      | |
      | |
      | |
      | |
      | |
      | |
      | |
      | |
      | |
  note: |
      | |
      | |
      | |
      | |
      | |
      | |
      | |
      | |
      | |
      | |
  note: Q1,Q2,Q3,Q4
  note: Q2,Q3
  note: Q4,Q1
  note: + Vdc -------------------------------
  note: - Vdc -------------------------------
  note: N -------
  note: |
      | |
      | |
      | |
      | |
      | |
      | |
      | |
      | |
      | |
      | |
  note: ---------- A
  note: --------[D-NN]---------
  note: --------[D_NP]---------
  note: |
      | |
      | [G4]
      | |
      | |
      | |
  note: |
      | |
      | [Q3]
      | |
      | |
  note: |
      | |
      | [Q2]
      | |
      | |
  note: |
      | |
      | |
      | [Q1]
      | |
      | |
  wt : Inport  PortDimensions=1
  sigma : Inport  Port=2  PortDimensions=1
  D_Alpha : Inport  Port=3  PortDimensions=1
  Constant1 : Constant  Value=[0 -pi]
  Constant2 : Constant  Value=2*pi
  Constant3 : Constant  Value=0
  Constant8 : Constant  Value=pi
  Constant9 : Constant  Value=pi
  Deg->Rad2 : Gain  Gain=0.5  SaturateOnIntegerOverflow=on  OutDataTypeStr=Inherit: Same as input  ParamDataTypeStr=Inherit: Same as input
  Deg->Rad3 : Gain  Gain=-1  SaturateOnIntegerOverflow=on  OutDataTypeStr=Inherit: Same as input  ParamDataTypeStr=Inherit: Same as input
  Gain3 : Gain  Gain=2  SaturateOnIntegerOverflow=on  OutDataTypeStr=Inherit: Same as input  ParamDataTypeStr=Inherit: Same as input
  Logical Operator : Logic
  Logical Operator2 : Logic  Operator=NOT
  Math Function : Math  Operator=mod  SignedPower=on  SaturateOnIntegerOverflow=on
  Mux3 : Mux  Inputs=[2 2]
  Mux4 : Mux  Inputs=2
  Relational Operator : RelationalOperator  RndMeth=Nearest  InputSameDT=on
  Relational Operator1 : RelationalOperator  Operator=<  RndMeth=Nearest  InputSameDT=on
  Selector3 : Selector  InputPortWidth=4  IndexOptions=Index vector (dialog)  Indices=[4 1 2 3]  OutputSizes=1
  Sum{2,4..6} (4 alike) : Sum  InputSameDT=on  SaturateOnIntegerOverflow=on  OutDataTypeStr=Inherit: Same as first input
  Sum3 : Sum  Inputs=+-  InputSameDT=on  SaturateOnIntegerOverflow=on  OutDataTypeStr=Inherit: Same as first input
  Pulses : Outport
  wires:
  Constant2/1 -> Math Function/2
  Sum5/1 -> Sum2/1  "theta"
  wt/1 -> Sum5/1  "wt"
  D_Alpha/1 -> Mux4/1, Deg->Rad3/1
  Deg->Rad3/1 -> Mux4/2
  Mux4/1 -> Sum5/2
  Math Function/1 -> Relational Operator/1, Relational Operator1/1
  Gain3/1 -> Sum6/1
  Selector3/1 -> Pulses/1
  Mux3/1 -> Selector3/1
  Logical Operator2/1 -> Mux3/2
  Logical Operator/1 -> Mux3/1, Logical Operator2/1
  Sum4/1 -> Math Function/1
  Sum2/1 -> Sum4/2
  Sum6/1 -> Relational Operator1/2
  Constant8/1 -> Sum6/2
  Deg->Rad2/1 -> Gain3/1, Sum4/1  "Beta"
  Sum3/1 -> Deg->Rad2/1
  sigma/1 -> Sum3/2
  Constant9/1 -> Sum3/1
  Relational Operator1/1 -> Logical Operator/2
  Relational Operator/1 -> Logical Operator/1
  Constant3/1 -> Relational Operator/2
  Constant1/1 -> Sum2/2

== system final_upfc_400kv_wavelet_windfarm_q/UPFC Controller/SH Control (STATCOM)/Firing Pulses Generator/Bridge 1D/Phase B ==
  note: |
      | |
      | |
      | [Q1]
      | |
      | |
  note: |
      | |
      | [Q2]
      | |
      | |
  note: |
      | |
      | [Q3]
      | |
      | |
  note: |
      | |
      | [G4]
      | |
      | |
      | |
  note: --------[D_NP]---------
  note: --------[D-NN]---------
  note: ---------- A
  note: |
      | |
      | |
      | |
      | |
      | |
      | |
      | |
      | |
      | |
      | |
  note: N -------
  note: - Vdc -------------------------------
  note: + Vdc -------------------------------
  note: Q4,Q1
  note: Q2,Q3
  note: Q1,Q2,Q3,Q4
  note: |
      | |
      | |
      | |
      | |
      | |
      | |
      | |
      | |
      | |
      | |
  note: |
      | |
      | |
      | |
      | |
      | |
      | |
      | |
      | |
      | |
      | |
  note: |
      | |
      | |
      | |
      | |
      | |
      | |
      | |
      | |
      | |
      | |
  note: Pulses timing
      | ===========
  note: Normal 180deg
      | Operation
  note: Normal 180deg
      | Operation
  note: Normal 180deg
      | Operation
  note: I--------------------------------I-----------------------------I--
  note: 0
  note: 180
  note: 360
  note: ******************
  note: ******************
  note: ********************************************
  note: ******************************************
  note: Q1
  note: Q2
  note: Q3
  note: Q4
  note: |
      | |
      | |
  note: |
      | |
      | |
  note: <--Sigma-->
  wt : Inport  PortDimensions=1
  sigma : Inport  Port=2  PortDimensions=1
  D_Alpha : Inport  Port=3  PortDimensions=1
  Constant1 : Constant  Value=[0 -pi]
  Constant2 : Constant  Value=2*pi
  Constant3 : Constant  Value=0
  Constant8 : Constant  Value=pi
  Constant9 : Constant  Value=pi
  Deg->Rad2 : Gain  Gain=0.5  SaturateOnIntegerOverflow=on  OutDataTypeStr=Inherit: Same as input  ParamDataTypeStr=Inherit: Same as input
  Deg->Rad3 : Gain  Gain=-1  SaturateOnIntegerOverflow=on  OutDataTypeStr=Inherit: Same as input  ParamDataTypeStr=Inherit: Same as input
  Gain3 : Gain  Gain=2  SaturateOnIntegerOverflow=on  OutDataTypeStr=Inherit: Same as input  ParamDataTypeStr=Inherit: Same as input
  Logical Operator : Logic
  Logical Operator2 : Logic  Operator=NOT
  Math Function : Math  Operator=mod  SignedPower=on  SaturateOnIntegerOverflow=on
  Mux3 : Mux  Inputs=[2 2]
  Mux4 : Mux  Inputs=2
  Relational Operator : RelationalOperator  RndMeth=Nearest  InputSameDT=on
  Relational Operator1 : RelationalOperator  Operator=<  RndMeth=Nearest  InputSameDT=on
  Selector3 : Selector  InputPortWidth=4  IndexOptions=Index vector (dialog)  Indices=[4 1 2 3]  OutputSizes=1
  Sum{2,4..6} (4 alike) : Sum  InputSameDT=on  SaturateOnIntegerOverflow=on  OutDataTypeStr=Inherit: Same as first input
  Sum3 : Sum  Inputs=+-  InputSameDT=on  SaturateOnIntegerOverflow=on  OutDataTypeStr=Inherit: Same as first input
  Pulses : Outport
  wires:
  Constant1/1 -> Sum2/2
  Constant3/1 -> Relational Operator/2
  Relational Operator/1 -> Logical Operator/1
  Relational Operator1/1 -> Logical Operator/2
  Constant9/1 -> Sum3/1
  sigma/1 -> Sum3/2
  Sum3/1 -> Deg->Rad2/1
  Deg->Rad2/1 -> Sum4/1, Gain3/1  "Beta"
  Constant8/1 -> Sum6/2
  Sum6/1 -> Relational Operator1/2
  Sum2/1 -> Sum4/2
  Sum4/1 -> Math Function/1
  Logical Operator/1 -> Logical Operator2/1, Mux3/1
  Logical Operator2/1 -> Mux3/2
  Mux3/1 -> Selector3/1
  Selector3/1 -> Pulses/1
  Gain3/1 -> Sum6/1
  Math Function/1 -> Relational Operator1/1, Relational Operator/1
  Mux4/1 -> Sum5/2
  Deg->Rad3/1 -> Mux4/2
  D_Alpha/1 -> Deg->Rad3/1, Mux4/1
  wt/1 -> Sum5/1  "wt"
  Sum5/1 -> Sum2/1  "theta"
  Constant2/1 -> Math Function/2

== system final_upfc_400kv_wavelet_windfarm_q/UPFC Controller/SH Control (STATCOM)/Firing Pulses Generator/Bridge 1D/Phase C ==
  note: <--Sigma-->
  note: |
      | |
      | |
  note: |
      | |
      | |
  note: Q4
  note: Q3
  note: Q2
  note: Q1
  note: ******************************************
  note: ********************************************
  note: ******************
  note: ******************
  note: 360
  note: 180
  note: 0
  note: I--------------------------------I-----------------------------I--
  note: Normal 180deg
      | Operation
  note: Normal 180deg
      | Operation
  note: Normal 180deg
      | Operation
  note: Pulses timing
      | ===========
  note: |
      | |
      | |
      | |
      | |
      | |
      | |
      | |
      | |
      | |
      | |
  note: |
      | |
      | |
      | |
      | |
      | |
      | |
      | |
      | |
      | |
      | |
  note: |
      | |
      | |
      | |
      | |
      | |
      | |
      | |
      | |
      | |
      | |
  note: Q1,Q2,Q3,Q4
  note: Q2,Q3
  note: Q4,Q1
  note: + Vdc -------------------------------
  note: - Vdc -------------------------------
  note: N -------
  note: |
      | |
      | |
      | |
      | |
      | |
      | |
      | |
      | |
      | |
      | |
  note: ---------- A
  note: --------[D-NN]---------
  note: --------[D_NP]---------
  note: |
      | |
      | [G4]
      | |
      | |
      | |
  note: |
      | |
      | [Q3]
      | |
      | |
  note: |
      | |
      | [Q2]
      | |
      | |
  note: |
      | |
      | |
      | [Q1]
      | |
      | |
  wt : Inport  PortDimensions=1
  sigma : Inport  Port=2  PortDimensions=1
  D_Alpha : Inport  Port=3  PortDimensions=1
  Constant1 : Constant  Value=[0 -pi]
  Constant2 : Constant  Value=2*pi
  Constant3 : Constant  Value=0
  Constant8 : Constant  Value=pi
  Constant9 : Constant  Value=pi
  Deg->Rad2 : Gain  Gain=0.5  SaturateOnIntegerOverflow=on  OutDataTypeStr=Inherit: Same as input  ParamDataTypeStr=Inherit: Same as input
  Deg->Rad3 : Gain  Gain=-1  SaturateOnIntegerOverflow=on  OutDataTypeStr=Inherit: Same as input  ParamDataTypeStr=Inherit: Same as input
  Gain3 : Gain  Gain=2  SaturateOnIntegerOverflow=on  OutDataTypeStr=Inherit: Same as input  ParamDataTypeStr=Inherit: Same as input
  Logical Operator : Logic
  Logical Operator2 : Logic  Operator=NOT
  Math Function : Math  Operator=mod  SignedPower=on  SaturateOnIntegerOverflow=on
  Mux3 : Mux  Inputs=[2 2]
  Mux4 : Mux  Inputs=2
  Relational Operator : RelationalOperator  RndMeth=Nearest  InputSameDT=on
  Relational Operator1 : RelationalOperator  Operator=<  RndMeth=Nearest  InputSameDT=on
  Selector3 : Selector  InputPortWidth=4  IndexOptions=Index vector (dialog)  Indices=[4 1 2 3]  OutputSizes=1
  Sum{2,4..6} (4 alike) : Sum  InputSameDT=on  SaturateOnIntegerOverflow=on  OutDataTypeStr=Inherit: Same as first input
  Sum3 : Sum  Inputs=+-  InputSameDT=on  SaturateOnIntegerOverflow=on  OutDataTypeStr=Inherit: Same as first input
  Pulses : Outport
  wires:
  Constant2/1 -> Math Function/2
  Sum5/1 -> Sum2/1  "theta"
  wt/1 -> Sum5/1  "wt"
  D_Alpha/1 -> Mux4/1, Deg->Rad3/1
  Deg->Rad3/1 -> Mux4/2
  Mux4/1 -> Sum5/2
  Math Function/1 -> Relational Operator/1, Relational Operator1/1
  Gain3/1 -> Sum6/1
  Selector3/1 -> Pulses/1
  Mux3/1 -> Selector3/1
  Logical Operator2/1 -> Mux3/2
  Logical Operator/1 -> Mux3/1, Logical Operator2/1
  Sum4/1 -> Math Function/1
  Sum2/1 -> Sum4/2
  Sum6/1 -> Relational Operator1/2
  Constant8/1 -> Sum6/2
  Deg->Rad2/1 -> Gain3/1, Sum4/1  "Beta"
  Sum3/1 -> Deg->Rad2/1
  sigma/1 -> Sum3/2
  Constant9/1 -> Sum3/1
  Relational Operator1/1 -> Logical Operator/2
  Relational Operator/1 -> Logical Operator/1
  Constant3/1 -> Relational Operator/2
  Constant1/1 -> Sum2/2

== system final_upfc_400kv_wavelet_windfarm_q/UPFC Controller/SH Control (STATCOM)/Firing Pulses Generator/Bridge 1Y /Phase A ==
  note: |
      | |
      | |
      | [Q1]
      | |
      | |
  note: |
      | |
      | [Q2]
      | |
      | |
  note: |
      | |
      | [Q3]
      | |
      | |
  note: |
      | |
      | [G4]
      | |
      | |
      | |
  note: --------[D_NP]---------
  note: --------[D-NN]---------
  note: ---------- A
  note: |
      | |
      | |
      | |
      | |
      | |
      | |
      | |
      | |
      | |
      | |
  note: N -------
  note: - Vdc -------------------------------
  note: + Vdc -------------------------------
  note: Q4,Q1
  note: Q2,Q3
  note: Q1,Q2,Q3,Q4
  note: |
      | |
      | |
      | |
      | |
      | |
      | |
      | |
      | |
      | |
      | |
  note: |
      | |
      | |
      | |
      | |
      | |
      | |
      | |
      | |
      | |
      | |
  note: |
      | |
      | |
      | |
      | |
      | |
      | |
      | |
      | |
      | |
      | |
  note: Pulses timing
      | ===========
  note: Normal 180deg
      | Operation
  note: Normal 180deg
      | Operation
  note: Normal 180deg
      | Operation
  note: I--------------------------------I-----------------------------I--
  note: 0
  note: 180
  note: 360
  note: ******************
  note: ******************
  note: ********************************************
  note: ******************************************
  note: Q1
  note: Q2
  note: Q3
  note: Q4
  note: |
      | |
      | |
  note: |
      | |
      | |
  note: <--Sigma-->
  wt : Inport  PortDimensions=1
  sigma : Inport  Port=2  PortDimensions=1
  D_Alpha : Inport  Port=3  PortDimensions=1
  Constant1 : Constant  Value=[0 -pi]
  Constant2 : Constant  Value=2*pi
  Constant3 : Constant  Value=0
  Constant8 : Constant  Value=pi
  Constant9 : Constant  Value=pi
  Deg->Rad2 : Gain  Gain=0.5  SaturateOnIntegerOverflow=on  OutDataTypeStr=Inherit: Same as input  ParamDataTypeStr=Inherit: Same as input
  Deg->Rad3 : Gain  Gain=-1  SaturateOnIntegerOverflow=on  OutDataTypeStr=Inherit: Same as input  ParamDataTypeStr=Inherit: Same as input
  Gain3 : Gain  Gain=2  SaturateOnIntegerOverflow=on  OutDataTypeStr=Inherit: Same as input  ParamDataTypeStr=Inherit: Same as input
  Logical Operator : Logic
  Logical Operator2 : Logic  Operator=NOT
  Math Function : Math  Operator=mod  SignedPower=on  SaturateOnIntegerOverflow=on
  Mux3 : Mux  Inputs=[2 2]
  Mux4 : Mux  Inputs=2
  Relational Operator : RelationalOperator  RndMeth=Nearest  InputSameDT=on
  Relational Operator1 : RelationalOperator  Operator=<  RndMeth=Nearest  InputSameDT=on
  Selector3 : Selector  InputPortWidth=4  IndexOptions=Index vector (dialog)  Indices=[4 1 2 3]  OutputSizes=1
  Sum{2,4..6} (4 alike) : Sum  InputSameDT=on  SaturateOnIntegerOverflow=on  OutDataTypeStr=Inherit: Same as first input
  Sum3 : Sum  Inputs=+-  InputSameDT=on  SaturateOnIntegerOverflow=on  OutDataTypeStr=Inherit: Same as first input
  Pulses : Outport
  wires:
  Constant1/1 -> Sum2/2
  Constant3/1 -> Relational Operator/2
  Relational Operator/1 -> Logical Operator/1
  Relational Operator1/1 -> Logical Operator/2
  Constant9/1 -> Sum3/1
  sigma/1 -> Sum3/2
  Sum3/1 -> Deg->Rad2/1
  Deg->Rad2/1 -> Sum4/1, Gain3/1  "Beta"
  Constant8/1 -> Sum6/2
  Sum6/1 -> Relational Operator1/2
  Sum2/1 -> Sum4/2
  Sum4/1 -> Math Function/1
  Logical Operator/1 -> Logical Operator2/1, Mux3/1
  Logical Operator2/1 -> Mux3/2
  Mux3/1 -> Selector3/1
  Selector3/1 -> Pulses/1
  Gain3/1 -> Sum6/1
  Math Function/1 -> Relational Operator1/1, Relational Operator/1
  Mux4/1 -> Sum5/2
  Deg->Rad3/1 -> Mux4/2
  D_Alpha/1 -> Deg->Rad3/1, Mux4/1
  wt/1 -> Sum5/1  "wt"
  Sum5/1 -> Sum2/1  "theta"
  Constant2/1 -> Math Function/2
